simulink model "MatLab6"  (Simulink 8.3)
settings: Solver=ode45  StartTime=0.0  StopTime=100  MaxStep=0.01  RelTol=1e-3
values from neighbouring files (symbols this model uses):
  A = [0 1  0              0 ... (first row only)    [MatLab4p.m]    (also in MatLab5p.m = [     0        1       0        0; MatLab6p.m = [     0        1       0        0; _Labs.m = [     0        1       0        0; q2.m = [0 1  0   0)
  Am = blkdiag(M,M)    [MatLab5p.m]    (also in MatLab6p.m; _Labs.m; q2.m = 1; questao2.m = 1)
  B = [0; 1/M; 0; -1/(M*L)]    [MatLab4p.m]    (also in MatLab5p.m = [ 0    0; MatLab6p.m = [ 0    0; _Labs.m = [ 0    0; q2.m = [  0)
  Bm = blkdiag(N,N)    [MatLab5p.m]    (also in MatLab6p.m; _Labs.m; q2.m = N; questao2.m = N)
  C = [1 0 0 0]    [MatLab4p.m]    (also in MatLab5p.m = [1 0 0 0; MatLab6p.m = [1 0 0 0; _Labs.m = [1 0 0 0; q2.m)
  Dsim = zeros(4,1)    [MatLab4p.m]    (also in MatLab5p.m = zeros(4,2); MatLab6p.m = zeros(4,2); _Labs.m = zeros(4,2); q2.m)
  K = place(A,B,[-2 -2.05 -2.1 -2.15])    [MatLab4p.m]    (also in MatLab5p.m = Ka(:,1:4); MatLab6p.m = Ka(:,1:4); _Labs.m = Ka(:,1:4); q2.m = Ka(:,1:4))
  Km = Ka(:,5:10)    [MatLab5p.m]    (also in MatLab6p.m; _Labs.m; q2.m = Ka(5); questao2.m = Ka(:,5:7))
  L = (place(A',C',[-6 -6.05 -6.1 -6.15]))'    [MatLab4p.m]    (also in MatLab6p.m = H'; _Labs.m = H'; q2.m = H'; questao2.m = H')
  x0 = [0 0 pi/4 0]    [MatLab4p.m]    (also in MatLab5p.m = [1 0.5 1 0.1]; MatLab6p.m = [1 2 0.8 -0.3]; _Labs.m = [1 2 0.8 -0.3]; q2.m = [0 0 pi/6 0])
  x0obs = [0.05 0 pi/5 0]    [MatLab4p.m]    (also in MatLab6p.m = [0 0 0 0]; _Labs.m = [0 0 0 0]; questao2.m = [0 0 0 0])
settings Model: Creator=hector  LastModifiedBy=hector
settings DataIOCC: SignalLoggingSaveFormat=Dataset
settings DebuggingCC: UnderspecifiedInitializationDetection=Simplified  StateNameClashWarn=none
settings GRTTargetCC: CombineOutputUpdateFcns=on  GRTInterface=off

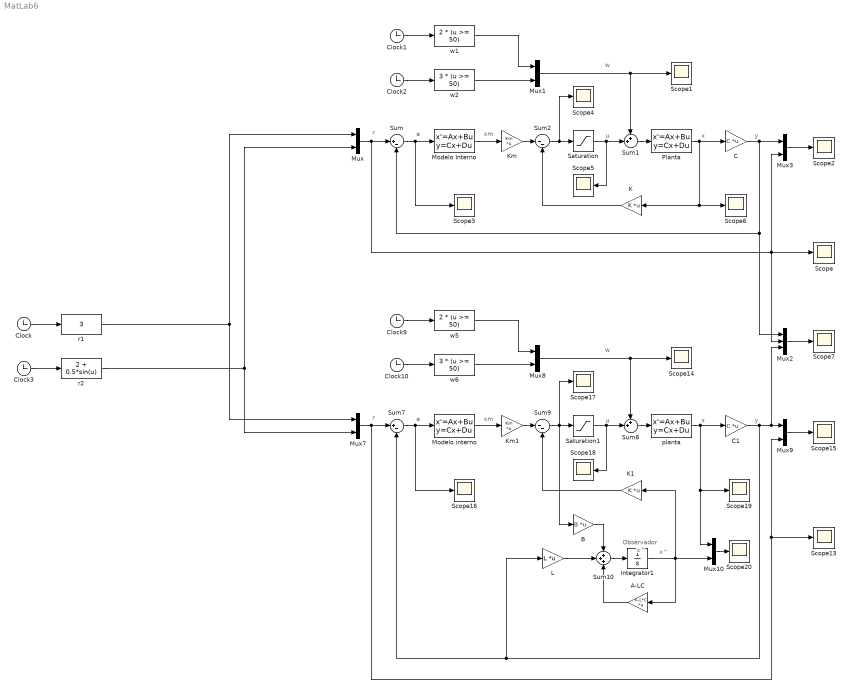
== system MatLab6 ==
  note: w
  note: u
  note: xm
  note: e
  note: r
  note: x
  note: y
  note: w
  note: u
  note: xm
  note: e
  note: r
  note: x
  note: y
  note: Observador
  note: x^
  note: x^
  A-LC : Gain  Gain=A-L*C  Multiplication=Matrix(K*u)
  B : Gain  Gain=B  Multiplication=Matrix(K*u)
  C : Gain  Gain=C  Multiplication=Matrix(K*u)
  C1 : Gain  Gain=C  Multiplication=Matrix(K*u)
  Clock{,1..3,9..10} (6 alike) : Clock
  Integrator1 : Integrator  InitialCondition=x0obs
  K : Gain  Gain=K  Multiplication=Matrix(K*u)
  K1 : Gain  Gain=K  Multiplication=Matrix(K*u)
  Km : Gain  Gain=Km  Multiplication=Matrix(K*u)
  Km1 : Gain  Gain=Km  Multiplication=Matrix(K*u)
  L : Gain  Gain=L  Multiplication=Matrix(K*u)
  Modelo Interno : StateSpace  A=Am  B=Bm  C=eye(6)  D=zeros(6,2)  X0=0
  Modelo interno : StateSpace  A=Am  B=Bm  C=eye(6)  D=zeros(6,2)  X0=0
  Mux{,1,3,7..10} (7 alike) : Mux  Inputs=2
  Mux2 : Mux  Inputs=3
  Planta : StateSpace  A=A  B=B  C=eye(4)  D=Dsim  X0=x0
  Saturation : Saturate  UpperLimit=20  LowerLimit=-20
  Saturation1 : Saturate  UpperLimit=20  LowerLimit=-20
  Scope{,1..7,13..20} (16 alike) : Scope
      Scope13 settings: SaveName=ScopeData13
      Scope14 settings: SaveName=ScopeData14
      Scope15 settings: YMin=1.5  YMax=4.5  SaveName=ScopeData15
      Scope16 settings: YMin=-0.035  YMax=0.0025  SaveName=ScopeData16
      Scope17 settings: YMin=-2.5  YMax=50  SaveName=ScopeData17
      Scope18 settings: YMin=1  YMax=6  SaveName=ScopeData18
      Scope19 settings: ShowLegends=on  YMin=-0.5  YMax=3.25  SaveName=ScopeData19
      Scope2 settings: YMin=1.9  YMax=3.3  SaveName=ScopeData2
      Scope20 settings: ShowLegends=on  YMin=-1.5  YMax=3.25  SaveName=ScopeData20
      Scope3 settings: YMin=-0.035  YMax=0.0025  SaveName=ScopeData3
      Scope4 settings: YMin=-2.5  YMax=50  SaveName=ScopeData4
      Scope5 settings: YMin=1  YMax=6  SaveName=ScopeData5
      Scope6 settings: ShowLegends=on  YMin=-0.5  YMax=3.25  SaveName=ScopeData6
      Scope7 settings: ShowLegends=on  YMin=1.4  YMax=3.8  SaveName=ScopeData7
  Sum : Sum  Inputs=|+-
  Sum1 : Sum  Inputs=++|
  Sum10 : Sum  Inputs=+++
  Sum2 : Sum  Inputs=|--
  Sum7 : Sum  Inputs=|+-
  Sum8 : Sum  Inputs=++|
  Sum9 : Sum  Inputs=|--
  planta : StateSpace  A=A  B=B  C=eye(4)  D=Dsim  X0=x0
  r1 : Fcn  Expr=3
  r2 : Fcn  Expr=2 + 0.5*sin(u)
  w1 : Fcn  Expr=2 * (u >= 50)
  w2 : Fcn  Expr=3 * (u >= 50)
  w5 : Fcn  Expr=2 * (u >= 50)
  w6 : Fcn  Expr=3 * (u >= 50)
  wires:
  Clock1/1 -> w1/1
  Sum/1 -> Modelo Interno/1, Scope3/1
  Sum1/1 -> Planta/1
  Clock2/1 -> w2/1
  r1/1 -> Mux7/1, Mux/1
  Clock/1 -> r1/1
  Clock3/1 -> r2/1
  r2/1 -> Mux7/2, Mux/2
  w1/1 -> Mux1/1
  w2/1 -> Mux1/2
  Mux1/1 -> Sum1/1, Scope1/1
  Planta/1 -> C/1, Scope6/1, K/1
  Mux3/1 -> Scope2/1
  Sum2/1 -> Saturation/1, Scope4/1
  Km/1 -> Sum2/1
  Modelo Interno/1 -> Km/1
  K/1 -> Sum2/2
  C/1 -> Mux3/1, Sum/2, Mux2/1
  Mux/1 -> Sum/1, Mux2/2, Scope/1, Mux3/2
  Saturation/1 -> Sum1/2, Scope5/1
  Clock9/1 -> w5/1
  Sum7/1 -> Modelo interno/1, Scope16/1
  Sum8/1 -> planta/1
  Clock10/1 -> w6/1
  w5/1 -> Mux8/1
  w6/1 -> Mux8/2
  Mux8/1 -> Sum8/1, Scope14/1
  planta/1 -> C1/1, Scope19/1, Mux10/1
  Mux9/1 -> Scope15/1
  Sum9/1 -> B/1, Saturation1/1, Scope17/1
  Km1/1 -> Sum9/1
  Modelo interno/1 -> Km1/1
  K1/1 -> Sum9/2
  C1/1 -> Mux2/3, Mux9/1, L/1, Sum7/2
  Mux7/1 -> Sum7/1, Scope13/1, Mux9/2
  Saturation1/1 -> Sum8/2, Scope18/1
  Sum10/1 -> Integrator1/1
  L/1 -> Sum10/2
  A-LC/1 -> Sum10/3
  Integrator1/1 -> Mux10/2, A-LC/1, K1/1
  B/1 -> Sum10/1
  Mux10/1 -> Scope20/1
  Mux2/1 -> Scope7/1
